simulink library "variant_6_WEC_Sim_Lib"  (R2015b)
settings: Solver=ode45  StartTime=0.0  StopTime=10.0  RelTol=1e-3
undefined symbols (not defined in the file): body, constraint, mooring, pto, simu, waves, X, Y, Z
libraries: nesl_utility x168, sm_lib x94, vrlib x12
(part 7 of 7)

== matlab function variant_6_WEC_Sim_Lib/Body Elements/Rigid Body/Hydrodynamic Body/Hydrostatic Restoring Force Calculation/Linear and Nonlinear Restoring Force Variant Subsystem/Nonlinear Hydrostatic Restoring Force/Diffarction and Excitation Forces1 ==
  data: x input; elv input; center input; f output; tnorm input; area input; rho input; g input; cg input; p output; dt input; dtFe input; t input
function [f,p]  = nonLinearBuoyancy(x,elv,center,tnorm,area,rho,g,cg,dt,dtFe,t)
% Function to calculate buoyancy force and moment on a triangulated surface
% NOTE: This function assumes that the STL file is imported with its CG at 0,0,0
persistent oldF 
persistent oldP

if isempty(oldF)
    [f,p] = calc_buoyancy(x,elv,center,tnorm,area,rho,g,cg);
    oldF  = f;
    oldP  = p;
else
    if mod(t, dtFe) < dt/2
        [f,p] = calc_buoyancy(x,elv,center,tnorm,area,rho,g,cg);
        oldF  = f;
        oldP  = p;
    else
        f  = oldF;
        p  = oldP;
    end
end
end


function [f,p] = calc_buoyancy(x,elv,center,tnorm,area,rho,g,cg)
% Function to apply translation and rotation and calculate forces

% Compute new tri coords after cog rotation and translation
center = rotateXYZ(center,[1 0 0],x(4));
center = rotateXYZ(center,[0 1 0],x(5));
center = rotateXYZ(center,[0 0 1],x(6));
center = offsetXYZ(center,x);
center = offsetXYZ(center,cg);
% Compute new normal vectors coords after cog rotation
tnorm = rotateXYZ(tnorm,[1 0 0],x(4));
tnorm = rotateXYZ(tnorm,[0 1 0],x(5));
tnorm = rotateXYZ(tnorm,[0 0 1],x(6));

% Calculate the hydrostatic forces
av = tnorm .* [area area area];
[f,p]=fHydrostatic(center,elv,x(1:3)+cg,av,rho,g); 
end

function verts = offsetXYZ(verts,x)
% Function to move the position vertices
verts(:,1) = verts(:,1) + x(1);
verts(:,2) = verts(:,2) + x(2);
verts(:,3) = verts(:,3) + x(3);
end

function xn = rotateXYZ(x,ax,t)
	% Function to rotate a point about an arbitrary axis
	% x: 3-componenet coordiantes
	% ax: axis about which to rotate (must be a vector length 1)
	% t: rotation angle
	% xn: new coordinates after rotation
	rotMat = zeros(3);
	rotMat(1,1) = ax(1)*ax(1)*(1-cos(t))    + cos(t);
	rotMat(1,2) = ax(2)*ax(1)*(1-cos(t))    + ax(3)*sin(t);
	rotMat(1,3) = ax(3)*ax(1)*(1-cos(t))    - ax(2)*sin(t);
	rotMat(2,1) = ax(1)*ax(2)*(1-cos(t))    - ax(3)*sin(t);
	rotMat(2,2) = ax(2)*ax(2)*(1-cos(t))    + cos(t);
	rotMat(2,3) = ax(3)*ax(2)*(1-cos(t))    + ax(1)*sin(t);
	rotMat(3,1) = ax(1)*ax(3)*(1-cos(t))    + ax(2)*sin(t);
	rotMat(3,2) = ax(2)*ax(3)*(1-cos(t))    - ax(1)*sin(t);
	rotMat(3,3) = ax(3)*ax(3)*(1-cos(t))    + cos(t);
	xn = x*rotMat;
end

function [f,p] = fHydrostatic(center,elv,instcg,av,rho,g)
% Function to calculate the force and moment about the cog due to hydrostatic pressure
f = zeros(6,1);

% Zeor out regions above the mean free surface
z=center(:,3); z((z-elv)>0)=0;

% Calculate the hydrostatic pressure at each triangle center
pressureVect = rho*g.*[-z -z -z].*-av;
p = rho*g.*-z;
% Compute force about cog
f(1:3) = sum(pressureVect);

tmp1 = ones(length(center(:,1)),1);
tmp2 = tmp1*instcg';
center2cgVec = center-tmp2;

f(4:6)= sum(cross(center2cgVec,pressureVect));
end

== matlab function variant_6_WEC_Sim_Lib/Body Elements/Rigid Body/Hydrodynamic Body/Wave Diffraction and Excitation Force Calculation/Linear Excitation Or diffraction/Linear Wave Diffraction Force Variant Subsystem/Irregular Wave Excitation Force/MATLAB Function ==
  data: A input; Fext output; w input; fExtRE input; fExtIM input; phaseRand input; dw input; time input
function Fext = fcn(A,w,fExtRE,fExtIM,phaseRand,dw,time)
%#codegen

persistent A1 B1 B11 C1 D1 D11 E1 E11

A1=bsxfun(@plus,w*time,pi/2);
B1= sin(bsxfun(@plus,A1,phaseRand));
B11 = sin(bsxfun(@plus,w*time,phaseRand));
C1 = sqrt(bsxfun(@times,A,dw));
D1 =bsxfun(@times,fExtRE,C1);
D11 = bsxfun(@times,fExtIM,C1);
E1 = bsxfun(@times,B1,D1);
E11 = bsxfun(@times,B11,D11);

Fext = sum(bsxfun(@minus,E1,E11));

== matlab function variant_6_WEC_Sim_Lib/Moorings/MoorDyn/Structure/Motion Sensor/Angle ==
  data: Q input; E output
function E  = EulerAngle(Q)
%#codegen
E=zeros(3,1);
E(1) = atan2( (2*(Q(1)*Q(2)+Q(3)*Q(4))), (1-2* (Q(2)^2+Q(3)^2) ) );
E(2) = asin( 2* (Q(1)*Q(3) - Q(4)*Q(2)));
E(3) = atan2( (2*(Q(1)*Q(4)+Q(2)*Q(3))), (1-2* (Q(3)^2+Q(4)^2) ) );

== matlab function variant_6_WEC_Sim_Lib/Moorings/MoorDyn/MoorDyn/MoorDyn/Triggered Subsystem/MATLAB Function ==
  data: X input; FLines output; XD input; Time input; CoupTime input
function FLines  = MoorDyn_matlab_FCN(X,XD,Time,CoupTime)

    FLines = zeros(1,6);
    coder.extrinsic('MoorDyn_caller');
    
    FLines = MoorDyn_caller(X,XD,Time-CoupTime,CoupTime);

== matlab function variant_6_WEC_Sim_Lib/Body Elements/Rigid Body/Hydrodynamic Body/Structure/Motion Sensor/Angle ==
  data: Q input; E output
function E  = EulerAngle(Q)
% Euler Angle Type II or Tait-Bryan Angle for sequence 321 or zyx (Nautical or Cardan angles).
% Yaw [-180,180], followed by pitch [-90,90], followed by roll [-180,180]
E = zeros(3,1);
E(1) = atan2((2*(Q(1)*Q(2)+Q(3)*Q(4))),(1-2*(Q(2)^2+Q(3)^2)));
E(2) = asin(2*(Q(1)*Q(3)-Q(4)*Q(2)));
E(3) = atan2((2*(Q(1)*Q(4)+Q(2)*Q(3))),(1-2*(Q(3)^2+Q(4)^2)));

== matlab function variant_6_WEC_Sim_Lib/Moorings/MooringMatrix/Structure/Motion Sensor/Angle ==
  data: Q input; E output
function E  = EulerAngle(Q)
%#codegen
E=zeros(3,1);
E(1) = atan2( (2*(Q(1)*Q(2)+Q(3)*Q(4))), (1-2* (Q(2)^2+Q(3)^2) ) );
E(2) = asin( 2* (Q(1)*Q(3) - Q(4)*Q(2)));
E(3) = atan2( (2*(Q(1)*Q(4)+Q(2)*Q(3))), (1-2* (Q(3)^2+Q(4)^2) ) );

== matlab function variant_6_WEC_Sim_Lib/Body Elements/Rigid Body/Hydrodynamic Body/Morrison Element and ViscousDampingForceCalculation/Morrison Element Variant Subsystem/Morrison Element On/Regular Wave Excitation Force/MorrisonElements/OrbitalVelocity/MATLAB Function ==
  data: u output; v output; disp input size=[1 3]; k input size=[1 1]; omega input size=[1 1]; waveAmp input size=[1 1]; theta input size=[1 1]; t input size=[1 1]; rampT input size=[1 1]; beta input size=[1 1]; h input size=[1 1]; g input size=[1 1]; w output size=[1 1]; xa output; ya output; za output
function [u,v,w,xa,ya,za] = calc_orbital_velocity(disp,k,omega,waveAmp,theta,t,rampT, beta, h, g)
%#codegen


[u,v,w,xa,ya,za] = orbital_velocity(disp,k,omega,waveAmp,theta,t,rampT, beta, h, g);

== matlab function variant_6_WEC_Sim_Lib/Body Elements/Rigid Body/Non-Hydro Body/Structure/Motion Sensor/Angle ==
  data: Q input; E output
function E  = EulerAngle(Q)
% Euler Angle Type II or Tait-Bryan Angle for sequence 321 or zyx (Nautical or Cardan angles).
% Yaw [-180,180], followed by pitch [-90,90], followed by roll [-180,180]
E = zeros(3,1);
E(1) = atan2( (2*(Q(1)*Q(2)+Q(3)*Q(4))), (1-2* (Q(2)^2+Q(3)^2) ) );
E(2) = asin( 2* (Q(1)*Q(3) - Q(4)*Q(2)));
E(3) = atan2( (2*(Q(1)*Q(4)+Q(2)*Q(3))), (1-2* (Q(3)^2+Q(4)^2) ) );

== matlab function variant_6_WEC_Sim_Lib/Body Elements/Rigid Body/Hydrodynamic Body/Morrison Element and ViscousDampingForceCalculation/Morrison Element Variant Subsystem/Morrison Element On/Irregular Wave Excitation Force/MorrisonElements/MorisonElementIrregular/MATLAB Function ==
  data: u output; v output; disp input size=[1 3]; k input size=[1 1]; omega input size=[1 1]; waveAmp input size=[1 1]; theta input size=[1 1]; t input size=[1 1]; rampT input size=[1 1]; beta input size=[1 1]; h input size=[1 1]; g input size=[1 1]; w output size=[1 1]; xa output; ya output; za output
function [u,v,w,xa,ya,za] = calc_orbital_velocity(disp,k,omega,waveAmp,theta,t,rampT, beta, h, g)
%#codegen


[u,v,w,xa,ya,za] = orbital_velocity(disp,k,omega,waveAmp,theta,t,rampT, beta, h, g);

== matlab function variant_6_WEC_Sim_Lib/Body Elements/Rigid Body/Hydrodynamic Body/Wave Diffraction and Excitation Force Calculation/Linear Excitation Or diffraction/Linear Wave Excitation Force Variant Subsystem/Irregular Wave Excitation Force/MATLAB Function ==
  data: A input; Fext output; w input; fExtRE input; fExtIM input; phaseRand input; dw input; time input
function Fext = fcn(A,w,fExtRE,fExtIM,phaseRand,dw,time)
%#codegen

persistent A1 B1 B11 C1 D1 D11 E1 E11

A1=bsxfun(@plus,w*time,pi/2);
B1= sin(bsxfun(@plus,A1,phaseRand));
B11 = sin(bsxfun(@plus,w*time,phaseRand));
C1 = sqrt(bsxfun(@times,A,dw));
D1 =bsxfun(@times,fExtRE,C1);
D11 = bsxfun(@times,fExtIM,C1);
E1 = bsxfun(@times,B1,D1);
E11 = bsxfun(@times,B11,D11);

Fext = sum(bsxfun(@minus,E1,E11));
